simulink model "DAQ9002"  (R2021a)
settings: Solver=FixedStepAuto  StartTime=0.0  StopTime=inf  RelTol=1e-3  EnableMultiTasking=on
undefined symbols (not defined in the file or in its folder): adrv9002, phy
libraries: simulink x2
settings Model: Creator=labuser  LastModifiedBy=labuser
settings SolverCC: PositivePriorityOrder=on
settings OptimizationCC: DefaultParameterBehavior=Inlined  EnhancedBackFolding=on  PassReuseOutputArgsThreshold=0  MaxStackSize=64  OptimizeBlockOrder=speed  DifferentSizesBufferReuse=on  OptimizationCustomize=off
settings DebuggingCC: ParameterTunabilityLossMsg=error
settings SFSimCC: MATLABDynamicMemAlloc=off
settings RTWCC: Description=Simulink Desktop Real-Time  SystemTargetFile=sldrt.tlc  TemplateMakefile=sldrt.tmf  Toolchain=ARM Development Studio Altera Edition (DS-5 AE)  RTWCompilerOptimization=on
settings CodeAppCC: ForceParamTrailComments=on  MaxIdLength=95  OperatorAnnotations=on
settings SimulinkDesktopRealTimeCC: TargetPreCompLibLocation=C:\Program Files\MATLAB\R2021a\toolbox\sldrt\lib\win64  TargetLangStandard=C89/C90 (ANSI)

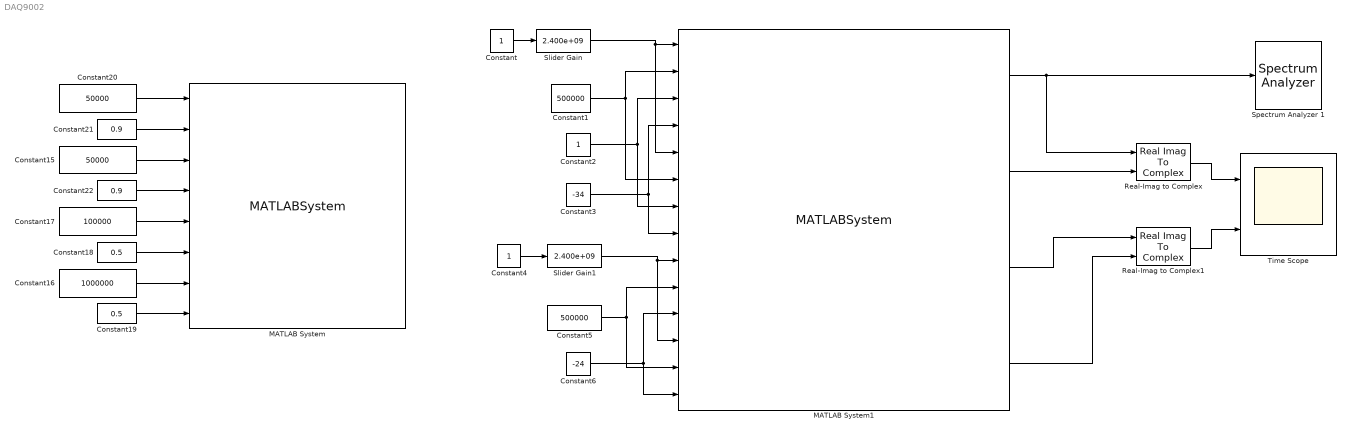
== system DAQ9002 ==
  Constant : Constant
  Constant1 : Constant  Value=500000
  Constant15 : Constant  Value=50000
  Constant16 : Constant  Value=1000000
  Constant17 : Constant  Value=100000
  Constant18 : Constant  Value=0.5
  Constant19 : Constant  Value=0.5
  Constant2 : Constant
  Constant20 : Constant  Value=50000
  Constant21 : Constant  Value=0.9
  Constant22 : Constant  Value=0.9
  Constant3 : Constant  Value=-34
  Constant4 : Constant
  Constant5 : Constant  Value=500000
  Constant6 : Constant  Value=-24
  MATLAB System : MATLABSystem  System=iio_sys_obj  ip_address=10.126.202.153  dev_name=axi-adrv9002-tx-lpc  in_ch_no=0  in_ch_size=8192  out_ch_no=0  out_ch_size=8192  SimulateUsing=Interpreted execution
      mask Type: iio_sys_obj
      mask Display:
      | disp('axi-adrv9002-tx-lpc');
      | port_label('input',1,'channel = TX1_I_F1_Freq');
      | port_label('input',2,'channel = TX1_I_F1_Scale');
      | port_label('input',3,'channel = TX1_Q_F1_Freq');
      | port_label('input',4,'channel = TX1_Q_F1_Scale');
      | port_label('input',5,'channel = TX2_I_F1_Freq');
      | port_label('input',6,'channel = TX2_I_F1_Scale');
      | port_label('input',7,'channel = TX2_Q_F1_Freq');
      | port_label('input',8,'channel = TX2_Q_F1_Scale');
  MATLAB System1 : MATLABSystem  System=iio_sys_obj  ip_address=10.126.202.153  dev_name=adrv9002-phy  in_ch_no=0  in_ch_size=8192  out_ch_no=4  out_ch_size=8192  SimulateUsing=Interpreted execution
      mask Type: iio_sys_obj
      mask Display:
      | disp('adrv9002-phy');
      | port_label('input',1,'channel = RX1_LO_FREQ');
      | port_label('input',2,'channel = RX1_RF_BANDWIDTH');
      | port_label('input',3,'channel = RX1_GAIN_MODE');
      | port_label('input',4,'channel = RX1_GAIN');
      | port_label('input',5,'channel = RX2_LO_FREQ');
      | port_label('input',6,'channel = RX2_RF_BANDWIDTH');
      | port_label('input',7,'channel = RX2_GAIN_MODE');
      | port_label('input',8,'channel = RX2_GAIN');
      | port_label('input',9,'channel = TX1_LO_FREQ');
      | port_label('input',10,'channel = TX1_RF_BANDWIDTH');
      | port_label('input',11,'channel = TX1_GAIN');
      | port_label('input',12,'channel = TX2_LO_FREQ');
      | port_label('input',13,'channel = TX2_RF_BANDWIDTH');
      | port_label('input',14,'channel = TX2_GAIN');
      | port_label('output',1,'DATA_OUT1');
      | port_label('output',2,'DATA_OUT2');
      | port_label('output',3,'DATA_OUT3');
      | port_label('output',4,'DATA_OUT4');
  Real-Imag to Complex : RealImagToComplex
  Real-Imag to Complex1 : RealImagToComplex
  Slider Gain : simulink/Math Operations/Slider Gain  gain=2.400e+09  low=0  high=2400000000
  Slider Gain1 : simulink/Math Operations/Slider Gain  gain=2.400e+09  low=0  high=2400000000
  Spectrum Analyzer 1 : SpectrumAnalyzer
  Time Scope : Scope  NumInputPorts=2
  wires:
  MATLAB System1/2 -> Real-Imag to Complex/2
  Slider Gain/1 -> MATLAB System1/5, MATLAB System1/1
  Constant/1 -> Slider Gain/1
  Constant2/1 -> MATLAB System1/3, MATLAB System1/7
  Constant1/1 -> MATLAB System1/6, MATLAB System1/2
  Constant3/1 -> MATLAB System1/4, MATLAB System1/8
  Constant4/1 -> Slider Gain1/1
  Slider Gain1/1 -> MATLAB System1/9, MATLAB System1/12
  Constant5/1 -> MATLAB System1/10, MATLAB System1/13
  MATLAB System1/1 -> Real-Imag to Complex/1, Spectrum Analyzer 1/1
  Constant6/1 -> MATLAB System1/11, MATLAB System1/14
  Constant20/1 -> MATLAB System/1
  Constant16/1 -> MATLAB System/7
  Constant17/1 -> MATLAB System/5
  Constant15/1 -> MATLAB System/3
  Constant21/1 -> MATLAB System/2
  Constant22/1 -> MATLAB System/4
  Constant18/1 -> MATLAB System/6
  Constant19/1 -> MATLAB System/8
  MATLAB System1/3 -> Real-Imag to Complex1/1
  MATLAB System1/4 -> Real-Imag to Complex1/2
  Real-Imag to Complex/1 -> Time Scope/1
  Real-Imag to Complex1/1 -> Time Scope/2
